simulink library "MyLibrary"  (R2024b)
settings: Solver=VariableStepAuto  StartTime=0.0  StopTime=10.0  RelTol=1e-3
values from neighbouring files (symbols this model uses):
  chg_ctrl_par = [Icc Vcv V_hys T_hys Kp_v_chg Ki_v_chg Kp_i_chg Ki_i_chg Ts_chg D_max_chg t_chg_on k_chg]    [init_paras.m]
  chg_ev = [0 Icc]    [init_paras.m]
  chg_par = [L_chg Voc Rint Ts_chg I_SIGN t_chg_on]    [init_paras.m]
  inj_amp = INJ.amp    [init_paras.m]
  inj_channel = INJ.channel    [init_paras.m]
  inj_duty = INJ.duty    [init_paras.m]
  inj_dwell = INJ.dwell    [init_paras.m]
  inj_f = INJ.f    [init_paras.m]
  inj_k = INJ.k    [init_paras.m]
  inj_period = INJ.period    [init_paras.m]
  inj_phase = INJ.phase    [init_paras.m]
  inj_shape = INJ.shape    [init_paras.m]
  inj_t_on = INJ.t_on    [init_paras.m]
  K_hall = INJ.K_hall    [init_paras.m]
  prot_thr = [300 450 65 355 25 2e-3 0.55]    [init_paras.m]
  Ts_chg = 10e-6    (= 1e-05)    [init_paras.m]
  Ts_Control = 1/Fc    [init_paras.m]
  Ts_Power = 50e-9    (= 5e-08)    [init_paras.m]    (also in run_benchmark.m = evalin('base','Ts_Power'))
  Vf = 0.6    [init_paras.m]
undefined symbols (not defined in the file or in its folder): Cs_fet, gcbh, Rs_fet, sps_rtmsupport
libraries: $bdroot x2, spsControlledCurrentSourceLib x1, spsDiodeModel x1, spsIdealSwitchModel x1
settings Model: Creator=Client  LastModifiedBy=chang
settings DebuggingCC: SaveWithParameterizedLinksMsg=none
settings RTWCC: GPUComputeCapability=3.5

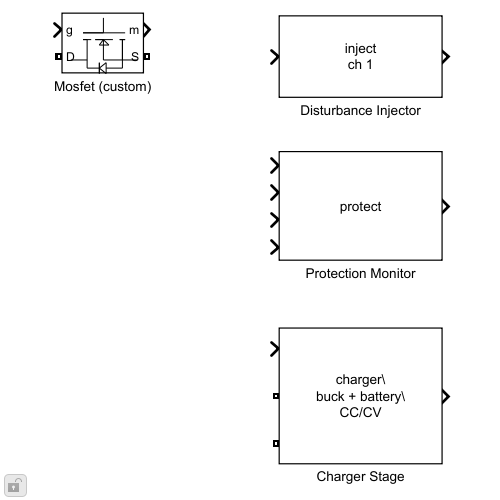
[thumbnail: Simulink's stored preview of the top-level diagram]
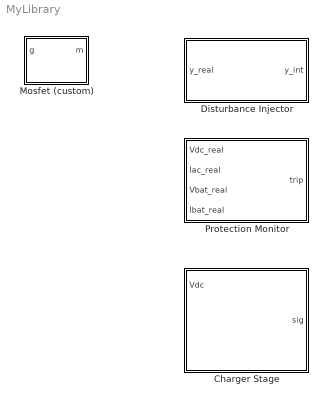
== system MyLibrary ==
  Charger Stage : Subsystem  mask(Charger Stage){}
      mask Display: disp('charger\\nbuck + battery\\nCC/CV')
  Disturbance Injector : Subsystem  mask(Disturbance Injector){ch_id=1, Ts_inj=Ts_Control, Ts_out=Ts_Power}
      mask prompts: ch_id "Channel id (1 Vdc 2 Vac 3 Iac 4 Vbat 5 Ibat)"; Ts_inj "Generator sample time"; Ts_out "Output sample time"
      mask Display: disp(sprintf('inject\\nch %d', ch_id))
  Mosfet (custom) : Subsystem  DialogController=POWERSYS.PowerSysDialog  LoadFcn=sps_rtmsupport('LoadFcn',gcbh);  StartFcn=sps_rtmsupport('StartFcn',gcbh);  StopFcn=sps_rtmsupport('StopFcn',gcbh);  mask(Custom FET){Ron=1e-3, Lon=0, Rd=1e-3, Vfd=Vf, IC=0, Rs=Rs_fet, Cs=Cs_fet, Measurements=on}
      mask prompts: Ron "FET resistance Ron (Ohms) :"; Lon "Internal diode inductance Lon (H) :"; Rd "Internal diode resistance Rd  (Ohms) :"; Vfd "Internal diode forward voltage Vf (V) :"; IC "Initial current Ic (A) :"; Rs "Snubber resistance Rs (Ohms) :"; Cs "Snubber capacitance Cs (F) :"; Measurements "Show measurement port"
      mask help: FET and internal diode in parallel with a series RC snubber circuit. When a gate signal is applied the MOSFET conducts and acts as a resistance (Ron) in both directions. If the gate signal falls to zero when current is negative, current is transferred to the antiparallel diode.
      mask init:
      | block = gcb;
      | [WantBlockChoice,Ts,X,Y,Ron] = powericon('SwitchesInit','MOSFET',block,Rs,Cs,Ron);
      | Csnubber  = Cs;
      settings: CopyFcn=sps_rtmsupport('CopyFcn',gcbh);  DeleteFcn=sps_rtmsupport('DeleteFcn',gcbh);  UndoDeleteFcn=sps_rtmsupport('UndoDeleteFcn',gcbh);  ModelCloseFcn=sps_rtmsupport('ModelCloseFcn',gcbh);  PreSaveFcn=sps_rtmsupport('PreSaveFcn',gcbh);  PostSaveFcn=sps_rtmsupport('PostSaveFcn',gcbh);  NameChangeFcn=sps_rtmsupport('NameChangeFcn',gcbh);  PreCopyFcn=sps_rtmsupport('PreCopyFcn',gcbh);  OpenFcn=sps_rtmsupport('OpenFcn',gcbh, 8);  CloseFcn=sps_rtmsupport('CloseFcn',gcbh);  PreDeleteFcn=sps_rtmsupport('PreDeleteFcn',gcbh);
      mask Help: helpview(psbhelp);
      mask Callback Ron: powericon('SwitchesEnables',gcb,'MOSFET');
      mask Display: plot(X.p1,Y.p1,X.p2,Y.p2,X.p3,Y.p3,X.p4,Y.p4,X.p5,Y.p5,X.p6,Y.p6,X.p7,Y.p7,X.p8,Y.p8)
  Protection Monitor : Subsystem  mask(Protection Monitor){}
      mask Display: disp('protect')

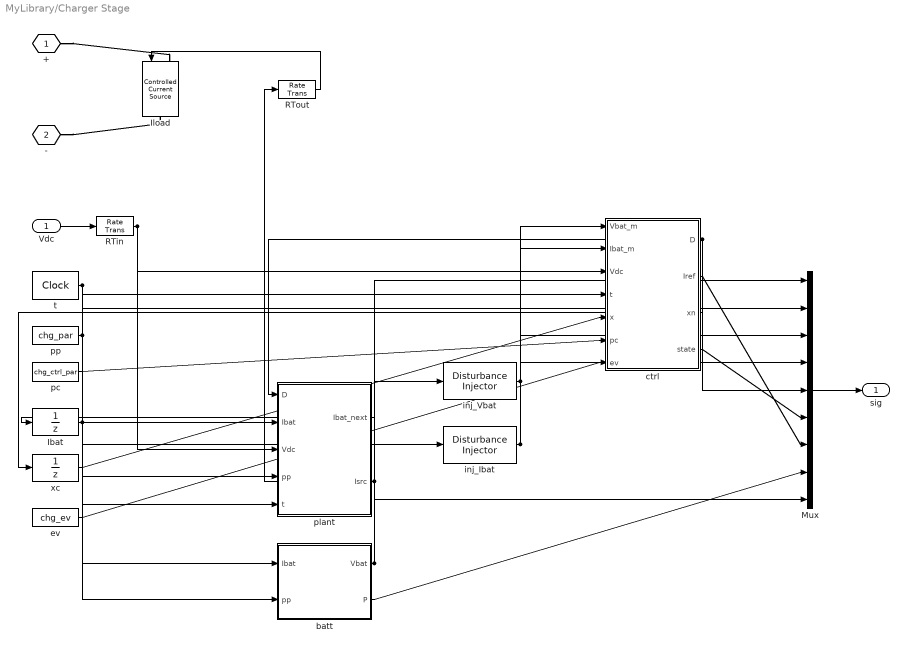
== system MyLibrary/Charger Stage ==
  Vdc : Inport
  Ibat : UnitDelay  SampleTime=Ts_chg  HasFrameUpgradeWarning=on
  Iload : spsControlledCurrentSourceLib/Controlled Current Source  Initialize=on  Source_Type=AC  Amplitude=0  Phase=0  Frequency=0  Measurements=None
  Mux : Mux  Inputs=9
  RTin : RateTransition  OutPortSampleTime=Ts_chg
  RTout : RateTransition  OutPortSampleTime=Ts_Power
  batt : MATLAB Function  TreatAsAtomicUnit=on
  ctrl : MATLAB Function  TreatAsAtomicUnit=on
  ev : Constant  Value=chg_ev
  inj_Ibat : $bdroot/Disturbance Injector  ch_id=5  Ts_inj=Ts_chg  Ts_out=Ts_chg
  inj_Vbat : $bdroot/Disturbance Injector  ch_id=4  Ts_inj=Ts_chg  Ts_out=Ts_chg
  pc : Constant  Value=chg_ctrl_par
  plant : MATLAB Function  TreatAsAtomicUnit=on
  pp : Constant  Value=chg_par
  t : DigitalClock  SampleTime=Ts_chg
  xc : UnitDelay  InitialCondition=zeros(1,4)  SampleTime=Ts_chg  HasFrameUpgradeWarning=on
  + : PMIOPort  Side=Left
  - : PMIOPort  Port=2  Side=Left
  sig : Outport
  wires:
  Vdc/1 -> RTin/1
  ctrl/1(D) -> plant/1(D), Mux/5
  Ibat/1 -> plant/2(Ibat), batt/1(Ibat), inj_Ibat/1, Mux/2
  RTin/1 -> plant/3(Vdc), ctrl/3(Vdc)
  pp/1 -> plant/4(pp), batt/2(pp)
  t/1 -> plant/5(t), ctrl/4(t)
  plant/1(Ibat_next) -> Ibat/1
  batt/1(Vbat) -> inj_Vbat/1, Mux/1
  inj_Vbat/1 -> ctrl/1(Vbat_m), Mux/3
  inj_Ibat/1 -> ctrl/2(Ibat_m), Mux/4
  xc/1 -> ctrl/5(x)
  pc/1 -> ctrl/6(pc)
  ev/1 -> ctrl/7(ev)
  ctrl/3(xn) -> xc/1
  plant/2(Isrc) -> RTout/1, Mux/9
  RTout/1 -> Iload/1
  ctrl/4(state) -> Mux/6
  ctrl/2(Iref) -> Mux/7
  batt/2(P) -> Mux/8
  Mux/1 -> sig/1
  connections:
  +/RConn1 -- Iload/LConn1
  -/RConn1 -- Iload/RConn1

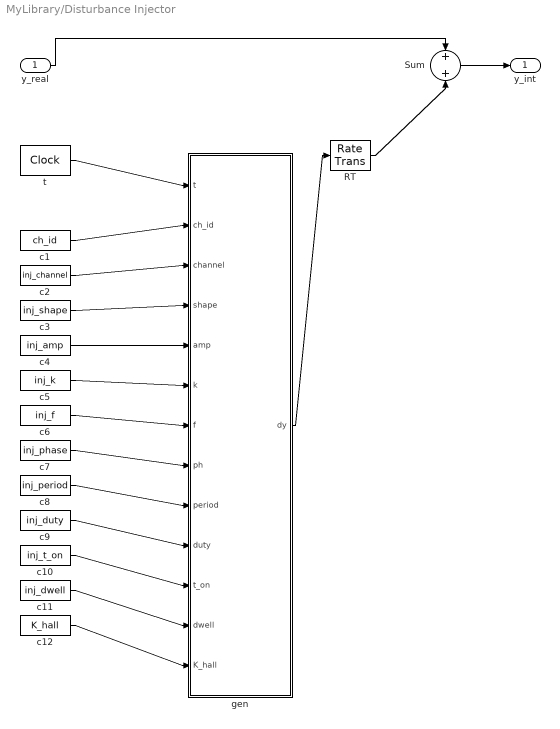
== system MyLibrary/Disturbance Injector ==
  y_real : Inport
  RT : RateTransition  OutPortSampleTime=Ts_out
  Sum : Sum
  c1 : Constant  Value=ch_id
  c10 : Constant  Value=inj_t_on
  c11 : Constant  Value=inj_dwell
  c12 : Constant  Value=K_hall
  c2 : Constant  Value=inj_channel
  c3 : Constant  Value=inj_shape
  c4 : Constant  Value=inj_amp
  c5 : Constant  Value=inj_k
  c6 : Constant  Value=inj_f
  c7 : Constant  Value=inj_phase
  c8 : Constant  Value=inj_period
  c9 : Constant  Value=inj_duty
  gen : MATLAB Function  TreatAsAtomicUnit=on
  t : DigitalClock  SampleTime=Ts_inj
  y_int : Outport
  wires:
  t/1 -> gen/1(t)
  c1/1 -> gen/2(ch_id)
  c2/1 -> gen/3(channel)
  c3/1 -> gen/4(shape)
  c4/1 -> gen/5(amp)
  c5/1 -> gen/6(k)
  c6/1 -> gen/7(f)
  c7/1 -> gen/8(ph)
  c8/1 -> gen/9(period)
  c9/1 -> gen/10(duty)
  c10/1 -> gen/11(t_on)
  c11/1 -> gen/12(dwell)
  c12/1 -> gen/13(K_hall)
  gen/1(dy) -> RT/1
  RT/1 -> Sum/2
  y_real/1 -> Sum/1
  Sum/1 -> y_int/1

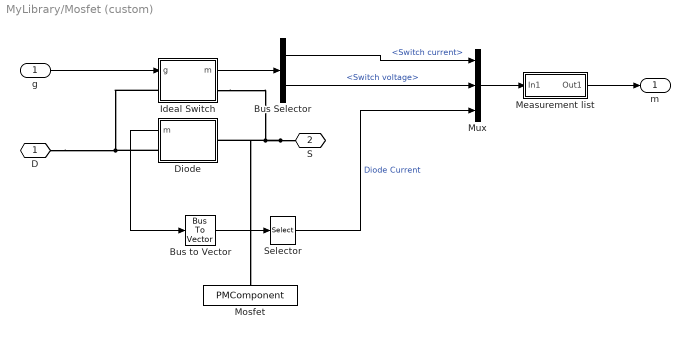
== system MyLibrary/Mosfet (custom) ==
  g : Inport
  Bus Selector : BusSelector  OutputSignals=Switch current,Switch voltage
  Bus to Vector : BusToVector
  Diode : Subsystem  DialogController=POWERSYS.PowerSysDialog  LoadFcn=sps_rtmsupport('LoadFcn',gcbh);  StartFcn=sps_rtmsupport('StartFcn',gcbh);  StopFcn=sps_rtmsupport('StopFcn',gcbh);  mask(Diode){Ron=Rd, Lon=Lon, Vf=Vfd, IC=0, UseSnubber=off, Rs=inf, Cs=0, Measurements=on}
      mask prompts: Ron "Resistance Ron (Ohms) :"; Lon "Inductance Lon (H) :"; Vf "Forward voltage Vf (V) :"; IC "Initial current Ic (A) :"; UseSnubber "Snubber"; Rs "Snubber resistance Rs (Ohms) :"; Cs "Snubber capacitance Cs (F) :"; Measurements "Show measurement port"
      mask help:
      | Implements a diode in parallel with a series RC snubber circuit.
      | In on-state the Diode model has an internal resistance (Ron) and inductance (Lon).
      | For most applications the internal inductance should be set to zero.
      | The Diode impedance is infinite in off-state mode.
      mask init:
      | block = gcb;
      | [WantBlockChoice,Ts,X,Y,Ron,Vf] = powericon('SwitchesInit','Diode',block,Rs,Cs,Ron,Vf);
      | powericon('SetInternalModels','set',block,WantBlockChoice);
      settings: CopyFcn=sps_rtmsupport('CopyFcn',gcbh); powericon('SwitchesCopyFcn','Diode',gcb)  DeleteFcn=sps_rtmsupport('DeleteFcn',gcbh);  UndoDeleteFcn=sps_rtmsupport('UndoDeleteFcn',gcbh);  ModelCloseFcn=sps_rtmsupport('ModelCloseFcn',gcbh);  PreSaveFcn=sps_rtmsupport('PreSaveFcn',gcbh);  PostSaveFcn=sps_rtmsupport('PostSaveFcn',gcbh);  NameChangeFcn=sps_rtmsupport('NameChangeFcn',gcbh);  PreCopyFcn=sps_rtmsupport('PreCopyFcn',gcbh);  OpenFcn=sps_rtmsupport('OpenFcn',gcbh, [5 8]);  CloseFcn=sps_rtmsupport('CloseFcn',gcbh);  PreDeleteFcn=sps_rtmsupport('PreDeleteFcn',gcbh);
      mask Help: helpview(psbhelp);
      mask Callback Ron: powericon('SwitchesEnables',gcb,'Diode');
      mask Callback Measurements:
      | powericon('OutputMCback',gcb);
      | %sps_rtmsupport('parametereditingmodes',gcbh, [5 8]);
      mask Display: plot(X.p1,Y.p1,X.p2,Y.p2,X.p3,Y.p3,X.p4,Y.p4,X.p5,Y.p5,X.p6,Y.p6)
  Ideal Switch : Subsystem  DialogController=POWERSYS.PowerSysDialog  LoadFcn=sps_rtmsupport('LoadFcn',gcbh);  StartFcn=sps_rtmsupport('StartFcn',gcbh);  StopFcn=sps_rtmsupport('StopFcn',gcbh);  mask(Ideal Switch){Ron=Ron, Lon=0, IC=0, Rs=Rs, Cs=Csnubber, Measurements=on}
      mask prompts: Ron "Internal resistance Ron (Ohms) :"; Lon "Inductance Lon (H) :"; IC "Initial state (0 for 'open', 1 for 'closed') :"; Rs "Snubber resistance Rs (Ohms) :"; Cs "Snubber capacitance Cs (F) :"; Measurements "Show measurement port"
      mask help:
      | Switch controlled by a gate signal in parallel with a series RC snubber circuit.
      | In on-state the Switch model has an internal resistance (Ron).
      |  In off-state this internal resistance is infinite.
      | The internal resistance must be greater than zero.
      | The switch model is on-state when the gate signal (g) is set to 1.
      mask init:
      | block = gcb;
      | [WantBlockChoice,Ts,X,Y,Ron] = powericon('SwitchesInit','Ideal Switch',block,Rs,Cs,Ron);
      | powericon('SetInternalModels','set',block,WantBlockChoice);
      settings: CopyFcn=sps_rtmsupport('CopyFcn',gcbh); powericon('SwitchesCopyFcn','Ideal Switch',gcb)  DeleteFcn=sps_rtmsupport('DeleteFcn',gcbh);  UndoDeleteFcn=sps_rtmsupport('UndoDeleteFcn',gcbh);  ModelCloseFcn=sps_rtmsupport('ModelCloseFcn',gcbh);  PreSaveFcn=sps_rtmsupport('PreSaveFcn',gcbh);  PostSaveFcn=sps_rtmsupport('PostSaveFcn',gcbh);  NameChangeFcn=sps_rtmsupport('NameChangeFcn',gcbh);  PreCopyFcn=sps_rtmsupport('PreCopyFcn',gcbh);  OpenFcn=sps_rtmsupport('OpenFcn',gcbh, 6);  CloseFcn=sps_rtmsupport('CloseFcn',gcbh);  PreDeleteFcn=sps_rtmsupport('PreDeleteFcn',gcbh);
      mask Help: helpview(psbhelp);
      mask Callback Ron: powericon('SwitchesEnables',gcb,'Ideal Switch');
      mask Callback Measurements: powericon('OutputMCback',gcb);
      mask Display: plot(X.p1,Y.p1,X.p2,Y.p2,X.p3,Y.p3,X.p4,Y.p4,X.p5,Y.p5)
  Measurement list : Subsystem
  Mosfet : PMComponent  PhysicalDomain=powersysdomain  LeftPortType=p1  RightPortType=p1  LConnTagsString=a  RConnTagsString=__new0  mask(InnerPowersysBlock){}
      mask Display: disp('SPS internal use\nDo not delete')
  Mux : Mux  Inputs=3
  Selector : Selector  InputPortWidth=2  IndexOptions=Index vector (dialog)  Indices=1  OutputSizes=1
  D : PMIOPort  Side=Left
  S : PMIOPort  Port=2  Side=Right
  m : Outport  VectorParamsAs1DForOutWhenUnconnected=off
  wires:
  Mux/1 -> Measurement list/1(In1)
  Selector/1 -> Mux/3  "Diode Current"
  Diode/1(m) -> Bus to Vector/1
  Ideal Switch/1(m) -> Bus Selector/1
  g/1 -> Ideal Switch/1(g)
  Measurement list/1(Out1) -> m/1
  Bus to Vector/1 -> Selector/1
  Bus Selector/2 -> Mux/2  "<Switch voltage>"
  Bus Selector/1 -> Mux/1  "<Switch current>"
  connections:
  Diode/RConn1 -- D/RConn1 -- Ideal Switch/LConn1
  S/RConn1 -- Diode/LConn1 -- Mosfet/LConn1 -- Ideal Switch/RConn1

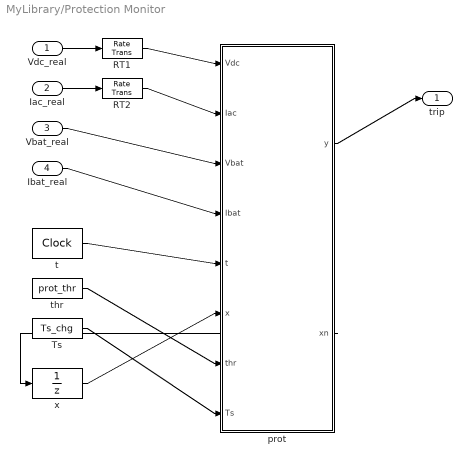
== system MyLibrary/Protection Monitor ==
  Vdc_real : Inport
  Iac_real : Inport  Port=2
  Vbat_real : Inport  Port=3
  Ibat_real : Inport  Port=4
  RT1 : RateTransition  OutPortSampleTime=Ts_chg
  RT2 : RateTransition  OutPortSampleTime=Ts_chg
  Ts : Constant  Value=Ts_chg
  prot : MATLAB Function  TreatAsAtomicUnit=on
  t : DigitalClock  SampleTime=Ts_chg
  thr : Constant  Value=prot_thr
  x : UnitDelay  InitialCondition=zeros(1,7)  SampleTime=Ts_chg  HasFrameUpgradeWarning=on
  trip : Outport
  wires:
  Vdc_real/1 -> RT1/1
  Iac_real/1 -> RT2/1
  RT1/1 -> prot/1(Vdc)
  RT2/1 -> prot/2(Iac)
  Vbat_real/1 -> prot/3(Vbat)
  Ibat_real/1 -> prot/4(Ibat)
  t/1 -> prot/5(t)
  x/1 -> prot/6(x)
  thr/1 -> prot/7(thr)
  Ts/1 -> prot/8(Ts)
  prot/1(y) -> trip/1
  prot/2(xn) -> x/1

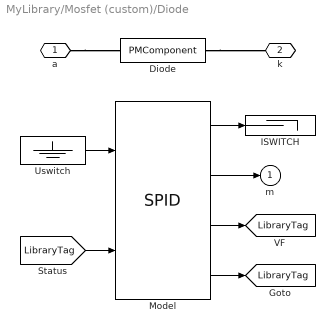
== system MyLibrary/Mosfet (custom)/Diode ==
  Diode : PMComponent  PhysicalDomain=powersysdomain  LeftPortType=p1  RightPortType=p1  LConnTagsString=a  RConnTagsString=__new0  mask(InnerPowersysBlock){}
      mask Display: disp('SPS internal use\nDo not delete')
  ISWITCH : Terminator
  Model : spsDiodeModel/SPID  SystemSampleTime=-1  VariantActivationTime=update diagram  Latency=0  AutoFrameSizeCalculation=off
  Uswitch : Ground
  a : PMIOPort  Side=Left
  k : PMIOPort  Port=2  Side=Right
  m : Outport  VectorParamsAs1DForOutWhenUnconnected=off
  tag scope: LibraryTag=global
  wires:
  Model/2 -> m/1
  [LibraryTag] -> Model/2
  Model/3 -> [LibraryTag]
  Model/4 -> [LibraryTag]
  Model/1 -> ISWITCH/1
  Uswitch/1 -> Model/1
  connections:
  Diode/RConn1 -- k/RConn1
  a/RConn1 -- Diode/LConn1

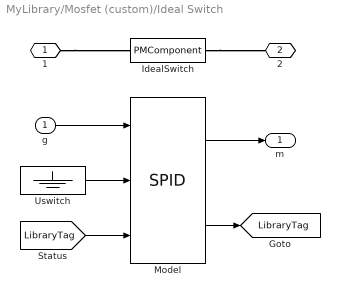
== system MyLibrary/Mosfet (custom)/Ideal Switch ==
  g : Inport
  IdealSwitch : PMComponent  PhysicalDomain=powersysdomain  LeftPortType=p1  RightPortType=p1  LConnTagsString=a  RConnTagsString=__new0  mask(InnerPowersysBlock){}
      mask Display: disp('SPS internal use\nDo not delete')
  Model : spsIdealSwitchModel/SPID  SystemSampleTime=-1  VariantActivationTime=update diagram  Latency=0  AutoFrameSizeCalculation=off
  Uswitch : Ground
  1 : PMIOPort  Side=Left
  2 : PMIOPort  Port=2  Side=Right
  m : Outport  VectorParamsAs1DForOutWhenUnconnected=off
  tag scope: LibraryTag=global
  wires:
  g/1 -> Model/1
  Model/1 -> m/1
  [LibraryTag] -> Model/3
  Model/2 -> [LibraryTag]
  Uswitch/1 -> Model/2
  connections:
  IdealSwitch/RConn1 -- 2/RConn1
  1/RConn1 -- IdealSwitch/LConn1

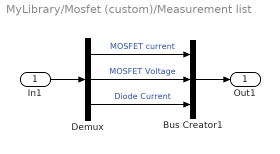
== system MyLibrary/Mosfet (custom)/Measurement list ==
  In1 : Inport
  Bus Creator1 : BusCreator  Inputs=3
  Demux : Demux  Outputs=[1,1,1]
  Out1 : Outport  VectorParamsAs1DForOutWhenUnconnected=off
  wires:
  In1/1 -> Demux/1
  Bus Creator1/1 -> Out1/1
  Demux/1 -> Bus Creator1/1  "MOSFET current"
  Demux/2 -> Bus Creator1/2  "MOSFET Voltage"
  Demux/3 -> Bus Creator1/3  "Diode Current"

== matlab function MyLibrary/Protection Monitor/prot ==
  data: Vdc input double size=1; y output double size=[1 2]; Iac input double size=1; Vbat input double size=1; Ibat input double size=1; t input double size=1; x input double size=[1 7]; thr input double size=[1 7]; Ts input double size=1; xn output double size=[1 7]
function [y, xn] = prot(Vdc, Iac, Vbat, Ibat, t, x, thr, Ts)
% x = [tUV tOV tOC tBOV tBOC trip t_trip]; thr = [UV OV OC BOV BOC hold t_arm]
% OC / BOC trip immediately, the others after |hold| seconds.  Armed from
% t_arm on, so the start-up inrush before the snapshot is ignored.
xn = x;
if t < thr(7), xn = zeros(1,7); y = [0 0]; return; end
cond = [Vdc < thr(1), Vdc > thr(2), abs(Iac) > thr(3), Vbat > thr(4), Ibat > thr(5)];
hold = [thr(6) thr(6) 0 thr(6) 0];
for i = 1:5
    if cond(i), xn(i) = x(i) + Ts; else, xn(i) = 0; end
end
if x(6) == 0
    for i = 1:5
        if cond(i) && xn(i) > hold(i), xn(6) = i; xn(7) = t; break; end
    end
end
y = xn(6:7);

== matlab function MyLibrary/Disturbance Injector/gen ==
  data: t input double size=1; dy output double size=1; ch_id input double size=1; channel input double size=[1 3]; shape input double size=[1 3]; amp input double size=[1 3]; k input double size=[1 3]; f input double size=[1 3]; ph input double size=[1 3]; period input double size=1; duty input double size=1; t_on input double size=1; dwell input double size=1; K_hall input double size=1
function dy = gen(t, ch_id, channel, shape, amp, k, f, ph, period, duty, t_on, dwell, K_hall)
% Equivalent measurement bias dy(t).  channel/shape/amp/k/f/ph are 1x3 so two
% channels can be disturbed at once (E-MUL-01) plus a noise slot; an entry
% with channel 0 is off.  Shape 7 = uniform white noise of amplitude amp
% (measurement noise, a benign negative sample for the detector).
dy = 0;
tau = t - t_on;
if tau < 0 || tau >= dwell, return; end
for i = 1:numel(channel)
    if channel(i) ~= ch_id, continue; end
    a = amp(i);
    switch shape(i)
        case 1, d = a;
        case 2, d = sign(a)*min(abs(a), k(i)*tau);
        case 3, d = a*sin(2*pi*f(i)*t + ph(i)*pi/180);
        case 4, x = mod(tau, period)/period; d = a*(1 - abs(2*x - 1));
        case 5, d = a*double(mod(tau, period) < duty*period);
        case 6, d = K_hall*(0.2 + 0.5*sin(2*pi*f(i)*t));
        case 7, d = a*(2*rand - 1);
        otherwise, d = 0;
    end
    dy = dy + d;
end

== matlab function MyLibrary/Charger Stage/plant ==
  data: D input double size=1; Ibat_next output double size=1; Ibat input double size=1; Vdc input double size=1; pp input double size=[1 6]; t input double size=1; Isrc output double size=1
function [Ibat_next, Isrc] = plant(D, Ibat, Vdc, pp, t)
% Averaged buck.  pp = [L_chg Voc Rint Ts_chg I_SIGN t_chg_on]
% Ibat is the inductor/battery current state (>= 0, diode conduction).
L = pp(1); Voc = pp(2); Rint = pp(3); Ts = pp(4); sgn = pp(5);
Vbat = Voc + Rint*Ibat;
Idc = D*Ibat;                      % lossless averaged input current
Isrc = sgn*Idc;
if t < pp(6)
    Ibat_next = 0;
else
    Ibat_next = Ibat + Ts/L*(D*Vdc - Vbat);
    if Ibat_next < 0, Ibat_next = 0; end
end

== matlab function MyLibrary/Charger Stage/batt ==
  data: Ibat input double size=1; Vbat output double size=1; pp input double size=[1 6]; P output double size=1
function [Vbat, P] = batt(Ibat, pp)
% Battery terminal voltage and charging power from the current state.
Vbat = pp(2) + pp(3)*Ibat;
P = Vbat*Ibat;

== matlab function MyLibrary/Charger Stage/ctrl ==
  data: Vbat_m input double size=1; D output double size=1; Ibat_m input double size=1; Vdc input double size=1; t input double size=1; x input double size=[1 4]; pc input double size=[1 12]; ev input double size=[1 2]; Iref output double size=1; xn output double size=[1 4]; state output double size=1
function [D, Iref, xn, state] = ctrl(Vbat_m, Ibat_m, Vdc, t, x, pc, ev)
% CC/CV charge controller.  x = [state tmr xv xi]  (0 CC, 1 CV)
% pc = [Icc Vcv Vhys Thys Kp_v Ki_v Kp_i Ki_i Ts Dmax t_on k_ramp]
% ev = [t_step Icc_new]: benign charging-current reference step (t_step <= 0: none)
Icc=pc(1); Vcv=pc(2); Vhys=pc(3); Thys=pc(4); Kpv=pc(5); Kiv=pc(6);
Kpi=pc(7); Kii=pc(8); Ts=pc(9); Dmax=pc(10); t_on=pc(11); kr=pc(12);
if ev(1) > 0 && t >= ev(1), Icc = ev(2); end
st = x(1); tmr = x(2); xv = x(3); xi = x(4);
Iramp = min(Icc, max(0, (t - t_on)*kr));
% --- state machine
if st == 0
    if Vbat_m >= Vcv, st = 1; tmr = 0; end
else
    if Vbat_m <= Vcv - Vhys, tmr = tmr + Ts; else, tmr = 0; end
    if tmr >= Thys, st = 0; tmr = 0; end
end
% --- outer voltage loop (CV only), preloaded to Iramp in CC
if st == 1
    ev = Vcv - Vbat_m;
    xv = xv + Kiv*ev*Ts;
    Iref = Kpv*ev + xv;
    if Iref > Iramp, Iref = Iramp; xv = min(xv, Iramp); end
    if Iref < 0,     Iref = 0;     xv = max(xv, 0); end
else
    Iref = Iramp; xv = Iramp;
end
% --- inner current loop with duty feed-forward
ei = Iref - Ibat_m;
xi = xi + Kii*ei*Ts;
Dff = Vbat_m / max(Vdc, 50);
D = Dff + Kpi*ei + xi;
if D > Dmax, D = Dmax; xi = xi - Kii*ei*Ts; end
if D < 0,    D = 0;    xi = xi - Kii*ei*Ts; end
if t < t_on, D = 0; xi = 0; end
xn = [st tmr xv xi];
state = st;
